simulink model "L8T1_HysteresisControlH_BridgeInverterUni"  (R2021a)
settings: Solver=VariableStepAuto  StartTime=0.0  StopTime=0.2  RelTol=1e-3
libraries: spsIGBTDiodeLib x4, spsVoltageMeasurementLib x2, spsACVoltageSourceLib x1, spsCurrentMeasurementLib x1, spsDCVoltageSourceLib x1, spsPLLLib x1, spsSeriesRLCBranchLib x1, spspowerguiLib x1
settings Model: Creator=hp  LastModifiedBy=hp

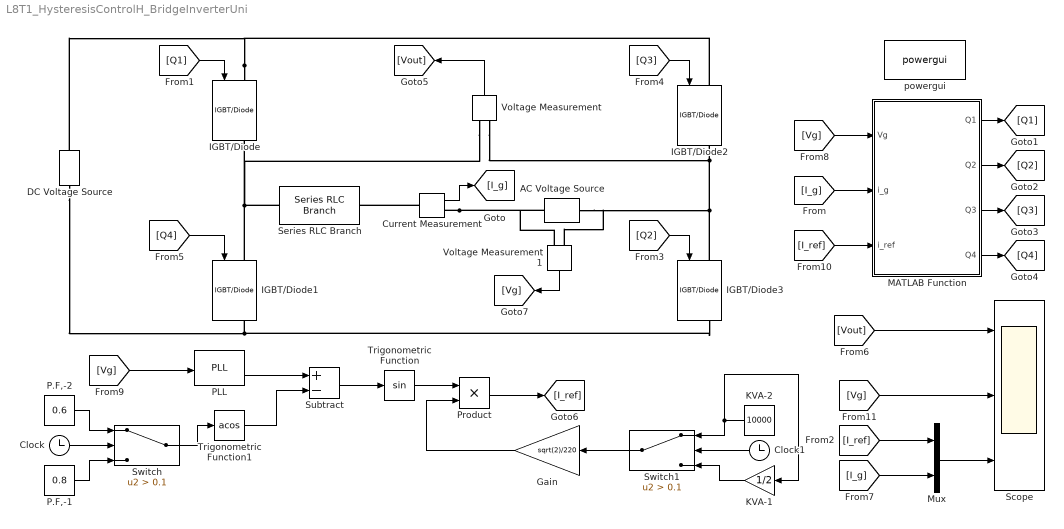
== system L8T1_HysteresisControlH_BridgeInverterUni ==
  AC Voltage Source : spsACVoltageSourceLib/AC Voltage Source  Amplitude=220*sqrt(2)  Phase=0  Frequency=50  SampleTime=0  Measurements=None  BusType=swing  Pref=10e3  Qref=0  Qmin=-inf  Qmax=+inf
  Clock : Clock
  Clock1 : Clock
  Current Measurement : spsCurrentMeasurementLib/Current Measurement  PhasorSimulation=off  OutputType=Complex  PSBequivalent=0
  DC Voltage Source : spsDCVoltageSourceLib/DC Voltage Source  Amplitude=400  Measurements=None
  Gain : Gain  Gain=sqrt(2)/220
  IGBT/Diode{,1..3} (4 alike) : spsIGBTDiodeLib/IGBT//Diode  Ron=1e-3  Rs=1e5  Cs=inf  Measurements=on
  KVA-1 : Gain  Gain=1/2
  KVA-2 : Constant  Value=10000
  MATLAB Function : MATLAB Function  TreatAsAtomicUnit=on
  Mux : Mux  Inputs=2
  P.F,-1 : Constant  Value=0.8
  P.F,-2 : Constant  Value=0.6
  PLL : spsPLLLib/PLL  Fmin=45  Par_Init=[0, 50]  ParK=[180, 3200, 1]  TcD=1e-4  MaxRateChangeFreq=12  FilterCutOffFreq=25  Ts=0  AGC=on
      settings: SourceProductBaseCode=PS
  Product : Product
  Scope : Scope  NumInputPorts=3
  Series RLC Branch : spsSeriesRLCBranchLib/Series RLC Branch  LConnTagsString=__new0  RConnTagsString=__new0  BranchType=RL  Resistance=0.1  Inductance=5e-3  SetiL0=off  InitialCurrent=0  Capacitance=1e-6  Setx0=off  InitialVoltage=0  Measurements=None
  Subtract : Sum  Inputs=+-
  Switch : Switch  Criteria=u2 > Threshold  Threshold=0.1
  Switch1 : Switch  Criteria=u2 > Threshold  Threshold=0.1
  Trigonometric Function : Trigonometry
  Trigonometric Function1 : Trigonometry  Operator=acos
  Voltage Measurement : spsVoltageMeasurementLib/Voltage Measurement  PhasorSimulation=off  OutputType=Complex  PSBequivalent=0
  Voltage Measurement1 : spsVoltageMeasurementLib/Voltage Measurement  PhasorSimulation=off  OutputType=Complex  PSBequivalent=0
  powergui : spspowerguiLib/powergui  Priority=1  SimulationMode=Discrete  SampleTime=50e-6  frequency=60  Iterations=50  frequencyindice=50  Pbase=100e6  ErrMax=1e-4  UnitsV=kV  UnitsW=MW  buscounter=0  FunctionMessages=off  echomessages=off  EnableUseOfTLC=off  CurrentSourceSwitches=off  DisableSnubberDevices=off  DisableRonSwitches=off  DisableVfSwitches=off  DisplayEquations=off  AutomaticDiscreteSolvers=off  SolverType=Tustin/Backward Euler (TBE)  Interpol=off  ExternalGateDelay=off  methode=off  Ts=100  x0status=blocks  SPID=on  SwTol=0  HookPort=off  NonlinearTolerance=1e-4  nMaxIteration=100  ContinueOnMaxIteration=off  RestoreLinks=warning  ResistiveCurrentMeasurement=off  Frange=[0:2:500]  Ylog=off  Xlog=on  ShowGrid=off  save=off  variable=ZData  structure=0  ZoomFFT=off  StartTime=0.0  cycles=1  DisplayStyle=1  fundamental=60  FreqAxis=off  MaxFrequency=1000  frequencyindicesteady=1  RmsSteady=1  display=off
  wires:
  [I_ref] -> MATLAB Function/3(i_ref)
  MATLAB Function/1(Q1) -> [Q1]
  [Vg] -> Scope/2
  [I_g] -> Mux/2
  [Vg] -> MATLAB Function/1(Vg)
  Current Measurement/1 -> [I_g]
  Voltage Measurement1/1 -> [Vg]
  [Q4] -> IGBT/Diode1/1
  [Vout] -> Scope/1
  MATLAB Function/3(Q3) -> [Q3]
  Voltage Measurement/1 -> [Vout]
  [I_ref] -> Mux/1
  MATLAB Function/2(Q2) -> [Q2]
  [Q1] -> IGBT/Diode/1
  Mux/1 -> Scope/3
  [Q3] -> IGBT/Diode2/1
  MATLAB Function/4(Q4) -> [Q4]
  [Q2] -> IGBT/Diode3/1
  [I_g] -> MATLAB Function/2(i_g)
  Clock1/1 -> Switch1/2
  Gain/1 -> Product/2
  Switch1/1 -> Gain/1
  Clock/1 -> Switch/2
  P.F,-1/1 -> Switch/3
  PLL/2 -> Subtract/1
  KVA-2/1 -> KVA-1/1, Switch1/1
  Trigonometric Function/1 -> Product/1
  Subtract/1 -> Trigonometric Function/1
  Product/1 -> [I_ref]
  KVA-1/1 -> Switch1/3
  Trigonometric Function1/1 -> Subtract/2
  P.F,-2/1 -> Switch/1
  [Vg] -> PLL/1
  Switch/1 -> Trigonometric Function1/1
  connections:
  IGBT/Diode/LConn1 -- DC Voltage Source/RConn1 -- IGBT/Diode2/LConn1
  Current Measurement/RConn1 -- AC Voltage Source/RConn1 -- Voltage Measurement1/LConn1
  Voltage Measurement/LConn2 -- IGBT/Diode2/RConn1 -- Voltage Measurement1/LConn2 -- AC Voltage Source/LConn1 -- IGBT/Diode3/LConn1
  Series RLC Branch/LConn1 -- IGBT/Diode1/LConn1 -- IGBT/Diode/RConn1 -- Voltage Measurement/LConn1
  DC Voltage Source/LConn1 -- IGBT/Diode1/RConn1 -- IGBT/Diode3/RConn1
  Current Measurement/LConn1 -- Series RLC Branch/RConn1

== matlab function L8T1_HysteresisControlH_BridgeInverterUni/MATLAB Function ==
  settings: updateMethod=DISCRETE
  data: Vg input; i_g input; Q1 output; i_ref input; Q2 output; Q3 output; Q4 output
function [Q1,Q2,Q3,Q4] = fcn(Vg,i_g,i_ref)
persistent s1 s2 s3 s4;
if isempty(s1)
    s1=0;
end
if isempty(s2)
    s2=0;
end
if isempty(s3)
    s3=0;
end
if isempty(s4)
    s4=0;
end
d=1;
e=i_g-i_ref;
if Vg>=0
    if e<=-d
        s1=1;   s2=1;   s3=0;    s4=0;
    elseif e>=d 
        s1=1;   s2=0;   s3=1;    s4=0;
    else 
        s1=s1;  s2=s2;  s3=s3;  s4=s4;
    end
else
    if e<=-d
        s1=1;   s2=0;   s3=1;    s4=0;
    elseif e>=d
        s1=0;   s2=0;   s3=1;    s4=1;
    else
        s1=s1;  s2=s2;  s3=s3;  s4=s4;
    end
   end
   Q1=s1;    Q2=s2;   Q3=s3;   Q4=s4;
end
